simulink model "test_SPHETModelAlgo"  (R2018b)
settings: Solver=ode1  StartTime=0.0  StopTime=10.0  FixedStep=0.1  RelTol=1e-3
undefined symbols (not defined in the file): sigbuilder_block
libraries: platooning_custom_blocks x1
settings Model: Creator=Aman-Home  LastModifiedBy=Aman-Home

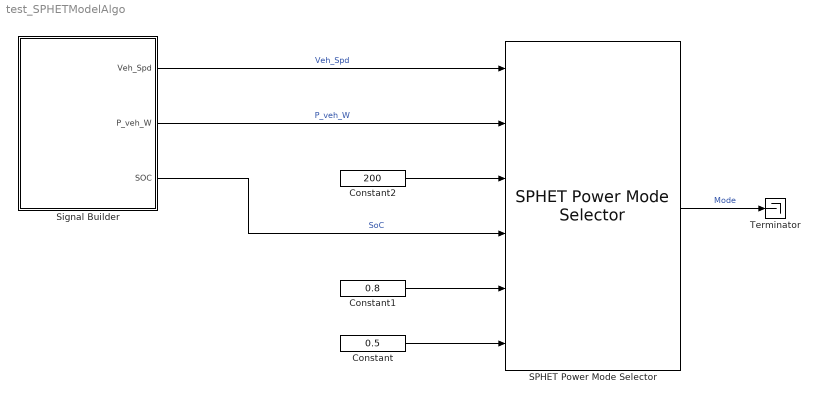
== system test_SPHETModelAlgo ==
  Constant : Constant  Value=0.5
  Constant1 : Constant  Value=0.8
  Constant2 : Constant  Value=200
  SPHET Power Mode Selector : platooning_custom_blocks/SPHET Power Mode Selector  SystemSampleTime=-1
  Signal Builder : Subsystem  Tag=STV Subsys  LoadFcn=sigbuilder_block('load');  StartFcn=sigbuilder_block('start');  StopFcn=sigbuilder_block('stop');  ClipboardFcn=sigbuilder_block('clipboard');  mask(Sigbuilder block){tuvar=[0:10]}
      mask help: Simulink:masks:SigbuilderBlock_MD
      mask init:
      | if ~strcmp(get_param(bdroot(gcbh),'SimulationStatus'),'stopped') tuvar = sigbuilder_block('maskInit'); end
      settings: CopyFcn=sigbuilder_block('copy');  DeleteFcn=sigbuilder_block('delete');  ModelCloseFcn=sigbuilder_block('modelClose');  PreSaveFcn=sigbuilder_block('preSave');  PauseFcn=sigbuilder_block('pause');  ContinueFcn=sigbuilder_block('continue');  NameChangeFcn=sigbuilder_block('namechange');  OpenFcn=sigbuilder_block('open',[712.5 234.75 550.5 399.75 ]);  CloseFcn=sigbuilder_block('close');
      mask Display: plot(0, 0, 100, 100,[2, 2, 32, 32, 2], [68, 8, 8, 68, 68],[32, 2], [38, 38], [32, 19, 2],[53, 60, 44], [32, 17, 17, 2],[16, 16, 31, 31]);txt = getActiveGroup(gcbh);text(2, 100, txt,'verticalAlignment', 'top');
  Terminator : Terminator
  wires:
  Constant/1 -> SPHET Power Mode Selector/6
  Constant1/1 -> SPHET Power Mode Selector/5
  Constant2/1 -> SPHET Power Mode Selector/3
  SPHET Power Mode Selector/1 -> Terminator/1  "Mode"
  Signal Builder/1(Veh_Spd) -> SPHET Power Mode Selector/1  "Veh_Spd"
  Signal Builder/2(P_veh_W) -> SPHET Power Mode Selector/2  "P_veh_W"
  Signal Builder/3(SOC) -> SPHET Power Mode Selector/4  "SoC"

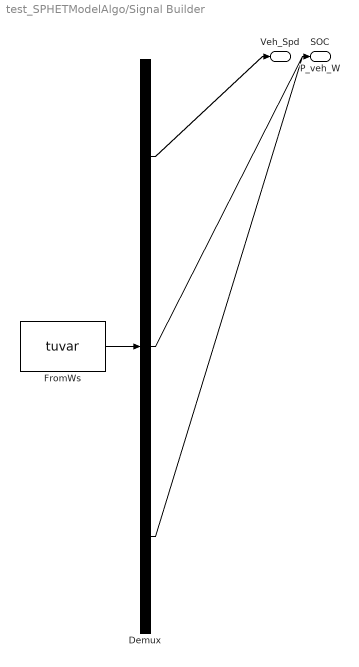
== system test_SPHETModelAlgo/Signal Builder ==
  Demux : Demux  Tag=STV Demux  Outputs=3
  FromWs : FromWorkspace  Tag=STV FromWs  VariableName=tuvar  SampleTime=0
      SigBuilderData=|
      | common.afterFinalStr = 'Extrapolate'
      | common.sampleTime = 0
      | dataSet.timeRange = [0 10]
      | dataSet.name = 'Group 1'
      | sbobj.Groups.Name = 'Group 1'
      | sbobj.Groups.Signals(1).Name = 'Veh_Spd'
      | sbobj.Groups.Signals(1).XData = [0 0.5 1 1.5 2 2.5 3 3.5 4 4.5 5 5.5 6 6.5 7 7.5 8 8.5 9 9.5 10]
      | sbobj.Groups.Signals(1).YData = [0 2 5 9 12 14 15 15 14 12 10 9 9 12 16 18 19 18 13 6 0]
      | sbobj.Groups.Signals(2).Name = 'P_veh_W'
      | sbobj.Groups.Signals(2).XData = [0 0.5 1 1.5 2 2.5 2.98 3.48 4 4.52 5 5.5 5.98 6.52 7 7.5 8 8.5 9 9.5 10]
      | sbobj.Groups.Signals(2).YData = [0 200 300 400 300 200 100 0 -100 -200 -200 -100 1 300 400 200 100 -100 -500 -700 -600]
      | sbobj.Groups.Signals(3).Name = 'SOC'
      | sbobj.Groups.Signals(3).XData = [0 0.5 0.951 1.5 2 2.55 3 3.5 4 4.5 5 5.5 6 6.6 7 7.55 8 8.5 9 9.55 10]
      | sbobj.Groups.Signals(3).YData = [0.6 0.58 0.55 0.51 0.48 0.46 0.46 0.46 0.47 0.48 0.5 0.51 0.52 0.51 0.49 0.47 0.47 0.47 0.49 0.51 0.51]
  Veh_Spd : Outport  Tag=STV Outport
  P_veh_W : Outport  Tag=STV Outport  Port=2
  SOC : Outport  Tag=STV Outport  Port=3
  wires:
  FromWs/1 -> Demux/1
  Demux/1 -> Veh_Spd/1
  Demux/2 -> P_veh_W/1
  Demux/3 -> SOC/1
